simulink model "Tiny_m8"  (R2020b)
settings: Solver=ode3  StartTime=0.0  StopTime=simTime  FixedStep=0.1  RelTol=1e-3  EnableMultiTasking=on
settings Model: Creator=aarrieta  LastModifiedBy=Xiao Ling
settings DataIOCC: ExternalInput=var  SaveFormat=Array  SignalLogging=off  DSMLogging=off  ReturnWorkspaceOutputs=off
settings OptimizationCC: LifeSpan=inf
settings DebuggingCC: UnderspecifiedInitializationDetection=Classic  MergeDetectMultiDrivingBlocksExec=none  SolverPrmCheckMsg=warning  StateNameClashWarn=warning  SFUnexpectedBacktrackingDiag=warning  SFNoUnconditionalDefaultTransitionDiag=warning  SFExecutionAtInitializationDiag=none  ArithmeticOperatorsInVariantConditions=warning
settings HardwareCC: ProdBitPerPointer=32  ProdBitPerSizeT=32  ProdBitPerPtrDiffT=32  ProdLargestAtomicFloat=None  ProdIntDivRoundTo=Undefined  ProdEndianess=Unspecified  ProdWordSize=32  ProdHWDeviceType=32-bit Generic
settings ModelReferenceCC: PropagateSignalLabelsOutOfModel=off
settings SFSimCC: SimUseLocalCustomCode=off  CustomCodeUndefinedFunction=UseInterfaceOnly
settings RTWCC: RTWUseLocalCustomCode=off
settings CodeAppCC: StateflowObjectComments=on
settings GRTTargetCC: TargetLangStandard=C89/C90 (ANSI)
settings ConfigComp: CovMetricSettings=dw  CovSaveCumulativeToWorkspaceVar=on  CovSaveSingleToWorkspaceVar=on  CovExternalEMLEnable=off

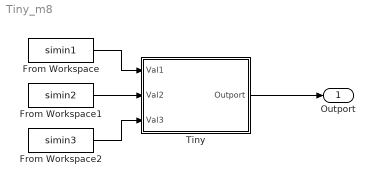
== system Tiny_m8 ==
  From Workspace : FromWorkspace  VariableName=simin1
  From Workspace1 : FromWorkspace  VariableName=simin2
  From Workspace2 : FromWorkspace  VariableName=simin3
  Tiny : Subsystem
  Outport : Outport
  wires:
  Tiny/1(Outport) -> Outport/1
  From Workspace/1 -> Tiny/1(Val1)
  From Workspace1/1 -> Tiny/2(Val2)
  From Workspace2/1 -> Tiny/3(Val3)

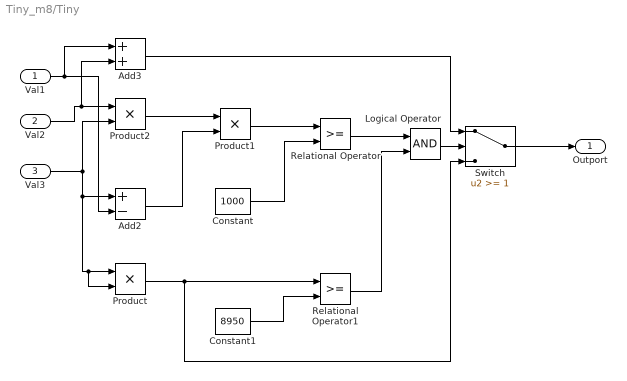
== system Tiny_m8/Tiny ==
  Val1 : Inport
  Val2 : Inport  Port=2
  Val3 : Inport  Port=3
  Add2 : Sum  Inputs=+-
  Add3 : Sum
  Constant : Constant  Value=1000
  Constant1 : Constant  Value=8950
  Logical Operator : Logic  AllPortsSameDT=off  OutDataTypeStr=boolean
  Product : Product
  Product1 : Product
  Product2 : Product
  Relational Operator : RelationalOperator  OutDataTypeStr=boolean  RndMeth=Nearest
  Relational Operator1 : RelationalOperator  OutDataTypeStr=boolean  RndMeth=Nearest
  Switch : Switch  Threshold=1
  Outport : Outport  VectorParamsAs1DForOutWhenUnconnected=off
  wires:
  Val3/1 -> Product2/2, Add2/1, Product/2, Product/1
  Val1/1 -> Add3/1, Add2/2
  Val2/1 -> Product2/1, Add3/2
  Product2/1 -> Product1/1
  Add2/1 -> Product1/2
  Product1/1 -> Relational Operator/1
  Product/1 -> Switch/3, Relational Operator1/1
  Constant/1 -> Relational Operator/2
  Constant1/1 -> Relational Operator1/2
  Relational Operator/1 -> Logical Operator/1
  Relational Operator1/1 -> Logical Operator/2
  Logical Operator/1 -> Switch/2
  Add3/1 -> Switch/1
  Switch/1 -> Outport/1
